simulink model "sim_SS_H2DF_2024a_GRU"  (R2024a)
settings: Solver=FixedStepAuto  StartTime=0.0  StopTime=4899  FixedStep=1  RelTol=1e-3  EnableMultiTasking=on
model workspace (MAT data in the model file):
  enable_IMEP_noise = 100
  enable_IMEP_offset = 1
values from neighbouring files (symbols this model uses):
  C2C_NMPC = init_C2C_NMPC_H2DF(C2C_NMPC.expdata)    [run_SS_H2DF_control.m]
undefined symbols (not defined in the file or in its folder): cost_length, horizon_length, y_ref_buf
libraries: matrix_library x3
(part 1 of 3)
settings Model: ExtModeTrigDuration=2  Creator=maxim  LastModifiedBy=winkler_a
settings SolverCC: PositivePriorityOrder=on
settings OptimizationCC: DefaultParameterBehavior=Inlined  EnhancedBackFolding=on  PassReuseOutputArgsAs=Individual arguments  ZeroExternalMemoryAtStartup=off  ZeroInternalMemoryAtStartup=off  MaxStackSize=64  OptimizeBlockOrder=speed  DifferentSizesBufferReuse=on  OptimizationCustomize=off  EfficientTunableParamExpr=on
settings DebuggingCC: ParameterTunabilityLossMsg=error
settings HardwareCC: ProdBitPerPointer=32  ProdBitPerSizeT=32  ProdBitPerPtrDiffT=32  ProdLargestAtomicInteger=Long  ProdLargestAtomicFloat=Double  ProdWordSize=32  ProdLongLongMode=on  ProdHWDeviceType=ARM Compatible->ARM Cortex
settings SFSimCC: SimUserSources=C2C_NMPC_model/C2C_NMPC_dyn_disc_phi_fun.c C2C_NMPC_model/C2C_NMPC_dyn_disc_phi_fun_jac.c C2C_NMPC_constraints/C2C_NMPC_constr_h_fun.c C2C_NMPC_constraints/C2C_NMPC_constr_h_fun_jac_uxt_zt.c C2C_NMPC_constraints/C2C_NMPC_constr_h_e_fun.c C2C_NMPC_constraints/C2C_NMPC_constr_h_e_fun_jac_uxt_zt.c acados_solver_sfunction_C2C_NMPC.c acados_solver_C2C_NMPC.c
settings SFSimCC: SimUserIncludeDirs=|
  | /include
  | /include/acados_c
  | /include/blasfeo/include
  | /include/hpipm/include
  | /lib
  | /c_generated_code
settings SFSimCC: SimUserLibraries=|
  | lib/libblasfeo.so
  | lib/libacados.so
  | lib/libhpipm.so
settings RTWCC: Description=Embedded Coder  SystemTargetFile=ert.tlc  TemplateMakefile=ert_default_tmf  RTWUseSimCustomCode=on  CustomSource=C2C_NMPC_model/C2C_NMPC_dyn_disc_phi_fun.c C2C_NMPC_model/C2C_NMPC_dyn_disc_phi_fun_jac.c C2C_NMPC_constraints/C2C_NMPC_constr_h_fun.c C2C_NMPC_constraints/C2C_NMPC_constr_h_fun_jac_uxt_zt.c C2C_NMPC_constraints/C2C_NMPC_constr_h_e_fun.c C2C_NMPC_constraints/C2C_NMPC_constr_h_e_fun_jac_uxt_zt.c acados_solver_sfunction_C2C_NMPC.c acados_solver_C2C_NMPC.c  Toolchain=GNU GCC Embedded Linux  BuildConfiguration=Faster Runs  GPUComputeCapability=3.5
settings RTWCC: CustomInclude=|
  | /include
  | /include/acados_c
  | /include/blasfeo/include
  | /include/hpipm/include
  | /lib
  | /c_generated_code
settings RTWCC: CustomLibrary=|
  | lib/libblasfeo.so
  | lib/libacados.so
  | lib/libhpipm.so
settings CodeAppCC: ForceParamTrailComments=on  IgnoreCustomStorageClasses=off  OperatorAnnotations=on  SimulinkDataObjDesc=on  SFDataObjDesc=on  InsertBlockDesc=on
settings ERTTargetCC: SupportContinuousTime=on  SupportNonInlinedSFcns=on  SupportVariableSizeSignals=on  ERTCustomFileTemplate=example_file_process.tlc

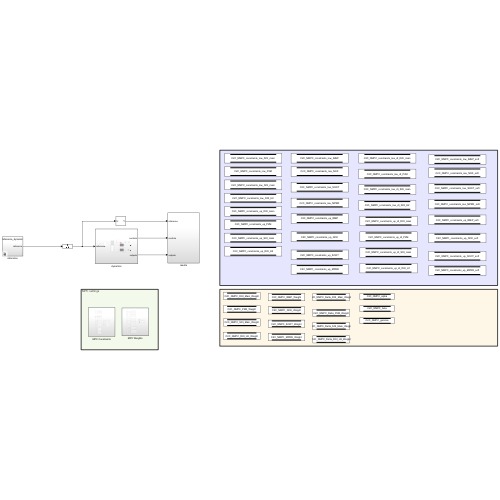
[thumbnail: Simulink's stored preview of the top-level diagram]
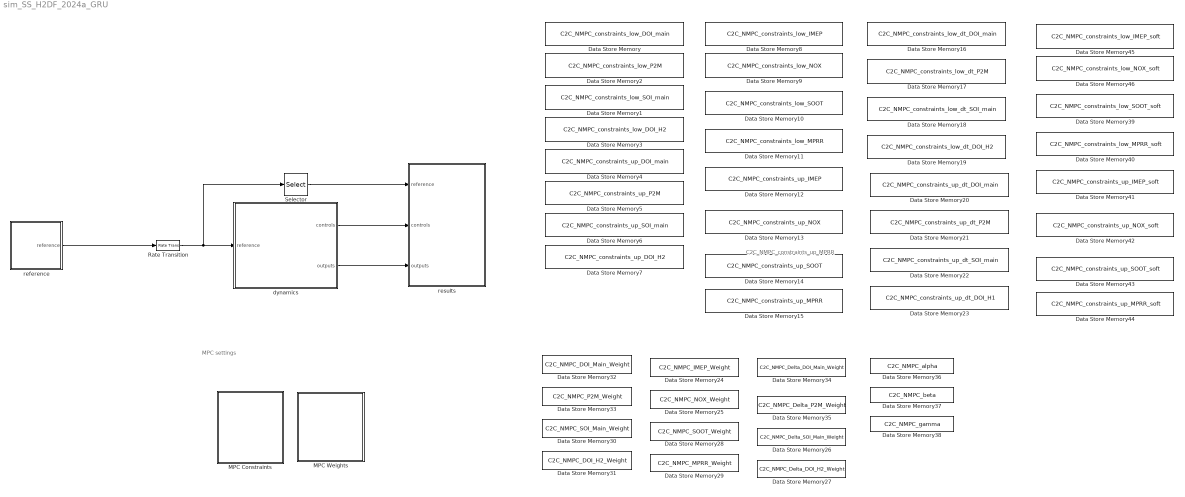
== system sim_SS_H2DF_2024a_GRU ==
  note: MPC settings
  note: C2C_NMPC_constraints_up_MPRR
  Data Store Memory : DataStoreMemory  DataStoreName=C2C_NMPC_constraints_low_DOI_main  WriteAfterWriteMsg=warning  ShowAdditionalParam=off
  Data Store Memory1 : DataStoreMemory  DataStoreName=C2C_NMPC_constraints_low_SOI_main  WriteAfterWriteMsg=warning  ShowAdditionalParam=off
  Data Store Memory10 : DataStoreMemory  DataStoreName=C2C_NMPC_constraints_low_SOOT  WriteAfterWriteMsg=warning  ShowAdditionalParam=off
  Data Store Memory11 : DataStoreMemory  DataStoreName=C2C_NMPC_constraints_low_MPRR  WriteAfterWriteMsg=warning  ShowAdditionalParam=off
  Data Store Memory12 : DataStoreMemory  DataStoreName=C2C_NMPC_constraints_up_IMEP  WriteAfterWriteMsg=warning  ShowAdditionalParam=off
  Data Store Memory13 : DataStoreMemory  DataStoreName=C2C_NMPC_constraints_up_NOX  WriteAfterWriteMsg=warning  ShowAdditionalParam=off
  Data Store Memory14 : DataStoreMemory  DataStoreName=C2C_NMPC_constraints_up_SOOT  WriteAfterWriteMsg=warning  ShowAdditionalParam=off
  Data Store Memory15 : DataStoreMemory  DataStoreName=C2C_NMPC_constraints_up_MPRR  WriteAfterWriteMsg=warning  ShowAdditionalParam=off
  Data Store Memory16 : DataStoreMemory  DataStoreName=C2C_NMPC_constraints_low_dt_DOI_main  WriteAfterWriteMsg=warning  ShowAdditionalParam=off
  Data Store Memory17 : DataStoreMemory  DataStoreName=C2C_NMPC_constraints_low_dt_P2M  WriteAfterWriteMsg=warning  ShowAdditionalParam=off
  Data Store Memory18 : DataStoreMemory  DataStoreName=C2C_NMPC_constraints_low_dt_SOI_main  WriteAfterWriteMsg=warning  ShowAdditionalParam=off
  Data Store Memory19 : DataStoreMemory  DataStoreName=C2C_NMPC_constraints_low_dt_DOI_H2  WriteAfterWriteMsg=warning  ShowAdditionalParam=off
  Data Store Memory2 : DataStoreMemory  DataStoreName=C2C_NMPC_constraints_low_P2M  WriteAfterWriteMsg=warning  ShowAdditionalParam=off
  Data Store Memory20 : DataStoreMemory  DataStoreName=C2C_NMPC_constraints_up_dt_DOI_main  WriteAfterWriteMsg=warning  ShowAdditionalParam=off
  Data Store Memory21 : DataStoreMemory  DataStoreName=C2C_NMPC_constraints_up_dt_P2M  WriteAfterWriteMsg=warning  ShowAdditionalParam=off
  Data Store Memory22 : DataStoreMemory  DataStoreName=C2C_NMPC_constraints_up_dt_SOI_main  WriteAfterWriteMsg=warning  ShowAdditionalParam=off
  Data Store Memory23 : DataStoreMemory  DataStoreName=C2C_NMPC_constraints_up_dt_DOI_H1  WriteAfterWriteMsg=warning  ShowAdditionalParam=off
  Data Store Memory24 : DataStoreMemory  DataStoreName=C2C_NMPC_IMEP_Weight  WriteAfterWriteMsg=warning  ShowAdditionalParam=off
  Data Store Memory25 : DataStoreMemory  DataStoreName=C2C_NMPC_NOX_Weight  WriteAfterWriteMsg=warning  ShowAdditionalParam=off
  Data Store Memory26 : DataStoreMemory  DataStoreName=C2C_NMPC_Delta_SOI_Main_Weight  WriteAfterWriteMsg=warning  ShowAdditionalParam=off
  Data Store Memory27 : DataStoreMemory  DataStoreName=C2C_NMPC_Delta_DOI_H2_Weight  WriteAfterWriteMsg=warning  ShowAdditionalParam=off
  Data Store Memory28 : DataStoreMemory  DataStoreName=C2C_NMPC_SOOT_Weight  WriteAfterWriteMsg=warning  ShowAdditionalParam=off
  Data Store Memory29 : DataStoreMemory  DataStoreName=C2C_NMPC_MPRR_Weight  WriteAfterWriteMsg=warning  ShowAdditionalParam=off
  Data Store Memory3 : DataStoreMemory  DataStoreName=C2C_NMPC_constraints_low_DOI_H2  WriteAfterWriteMsg=warning  ShowAdditionalParam=off
  Data Store Memory30 : DataStoreMemory  DataStoreName=C2C_NMPC_SOI_Main_Weight  WriteAfterWriteMsg=warning  ShowAdditionalParam=off
  Data Store Memory31 : DataStoreMemory  DataStoreName=C2C_NMPC_DOI_H2_Weight  WriteAfterWriteMsg=warning  ShowAdditionalParam=off
  Data Store Memory32 : DataStoreMemory  DataStoreName=C2C_NMPC_DOI_Main_Weight  WriteAfterWriteMsg=warning  ShowAdditionalParam=off
  Data Store Memory33 : DataStoreMemory  DataStoreName=C2C_NMPC_P2M_Weight  WriteAfterWriteMsg=warning  ShowAdditionalParam=off
  Data Store Memory34 : DataStoreMemory  DataStoreName=C2C_NMPC_Delta_DOI_Main_Weight  WriteAfterWriteMsg=warning  ShowAdditionalParam=off
  Data Store Memory35 : DataStoreMemory  DataStoreName=C2C_NMPC_Delta_P2M_Weight  WriteAfterWriteMsg=warning  ShowAdditionalParam=off
  Data Store Memory36 : DataStoreMemory  DataStoreName=C2C_NMPC_alpha  WriteAfterWriteMsg=warning  ShowAdditionalParam=off
  Data Store Memory37 : DataStoreMemory  DataStoreName=C2C_NMPC_beta  WriteAfterWriteMsg=warning  ShowAdditionalParam=off
  Data Store Memory38 : DataStoreMemory  DataStoreName=C2C_NMPC_gamma  WriteAfterWriteMsg=warning  ShowAdditionalParam=off
  Data Store Memory39 : DataStoreMemory  DataStoreName=C2C_NMPC_constraints_low_SOOT_soft  WriteAfterWriteMsg=warning  ShowAdditionalParam=off
  Data Store Memory4 : DataStoreMemory  DataStoreName=C2C_NMPC_constraints_up_DOI_main  WriteAfterWriteMsg=warning  ShowAdditionalParam=off
  Data Store Memory40 : DataStoreMemory  DataStoreName=C2C_NMPC_constraints_low_MPRR_soft  WriteAfterWriteMsg=warning  ShowAdditionalParam=off
  Data Store Memory41 : DataStoreMemory  DataStoreName=C2C_NMPC_constraints_up_IMEP_soft  WriteAfterWriteMsg=warning  ShowAdditionalParam=off
  Data Store Memory42 : DataStoreMemory  DataStoreName=C2C_NMPC_constraints_up_NOX_soft  WriteAfterWriteMsg=warning  ShowAdditionalParam=off
  Data Store Memory43 : DataStoreMemory  DataStoreName=C2C_NMPC_constraints_up_SOOT_soft  WriteAfterWriteMsg=warning  ShowAdditionalParam=off
  Data Store Memory44 : DataStoreMemory  DataStoreName=C2C_NMPC_constraints_up_MPRR_soft  WriteAfterWriteMsg=warning  ShowAdditionalParam=off
  Data Store Memory45 : DataStoreMemory  DataStoreName=C2C_NMPC_constraints_low_IMEP_soft  WriteAfterWriteMsg=warning  ShowAdditionalParam=off
  Data Store Memory46 : DataStoreMemory  DataStoreName=C2C_NMPC_constraints_low_NOX_soft  WriteAfterWriteMsg=warning  ShowAdditionalParam=off
  Data Store Memory5 : DataStoreMemory  DataStoreName=C2C_NMPC_constraints_up_P2M  WriteAfterWriteMsg=warning  ShowAdditionalParam=off
  Data Store Memory6 : DataStoreMemory  DataStoreName=C2C_NMPC_constraints_up_SOI_main  WriteAfterWriteMsg=warning  ShowAdditionalParam=off
  Data Store Memory7 : DataStoreMemory  DataStoreName=C2C_NMPC_constraints_up_DOI_H2  WriteAfterWriteMsg=warning  ShowAdditionalParam=off
  Data Store Memory8 : DataStoreMemory  DataStoreName=C2C_NMPC_constraints_low_IMEP  WriteAfterWriteMsg=warning  ShowAdditionalParam=off
  Data Store Memory9 : DataStoreMemory  DataStoreName=C2C_NMPC_constraints_low_NOX  WriteAfterWriteMsg=warning  ShowAdditionalParam=off
  MPC Constraints : Subsystem
  MPC Weights : Subsystem
  Rate Transition : RateTransition  Integrity=off  OutPortSampleTime=1
  Selector : Selector  InputPortWidth=C2C_NMPC.Dims.n_cost*3  IndexOptions=Index vector (dialog)  Indices=1:C2C_NMPC.Dims.n_cost  OutputSizes=1
  dynamics : Subsystem
  reference : Subsystem  Variant=on  VariantControlMode=label  VariantControl=Choice  LabelModeActiveChoice=reference_dynamic
  results : Subsystem
  wires:
  dynamics/2(outputs) -> results/3(outputs)
  Rate Transition/1 -> dynamics/1(reference), Selector/1
  dynamics/1(controls) -> results/2(controls)
  Selector/1 -> results/1(reference)
  reference/1(reference) -> Rate Transition/1

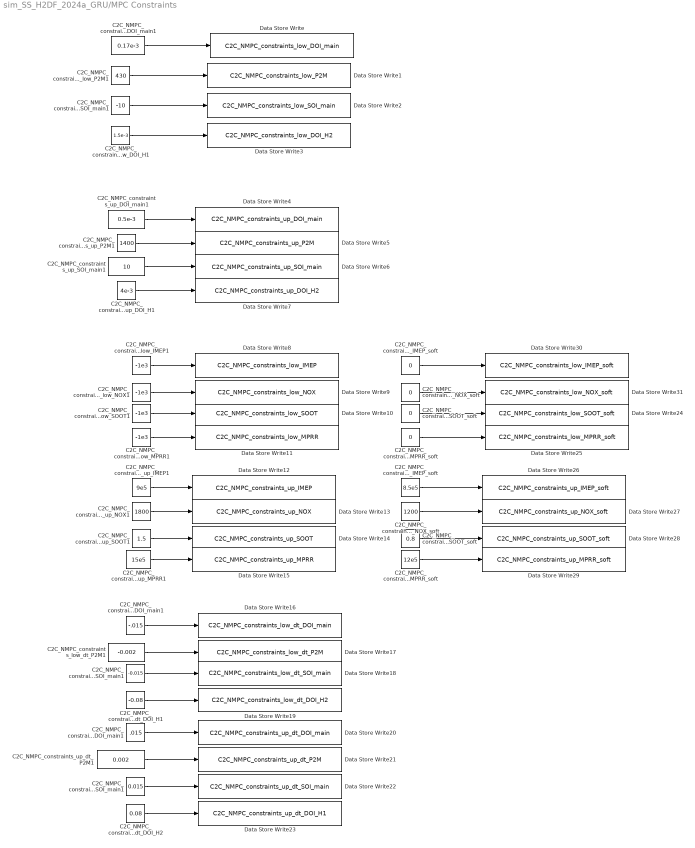
== system sim_SS_H2DF_2024a_GRU/MPC Constraints ==
  C2C_NMPC_constraints_low_DOI_H1 : Constant  Value=1.5e-3
  C2C_NMPC_constraints_low_DOI_main1 : Constant  Value=0.17e-3
  C2C_NMPC_constraints_low_IMEP1 : Constant  Value=-1e3
  C2C_NMPC_constraints_low_IMEP_soft : Constant  Value=0
  C2C_NMPC_constraints_low_MPRR1 : Constant  Value=-1e3
  C2C_NMPC_constraints_low_MPRR_soft : Constant  Value=0
  C2C_NMPC_constraints_low_NOX1 : Constant  Value=-1e3
  C2C_NMPC_constraints_low_NOX_soft : Constant  Value=0
  C2C_NMPC_constraints_low_P2M1 : Constant  Value=430
  C2C_NMPC_constraints_low_SOI_main1 : Constant  Value=-10
  C2C_NMPC_constraints_low_SOOT1 : Constant  Value=-1e3
  C2C_NMPC_constraints_low_SOOT_soft : Constant  Value=0
  C2C_NMPC_constraints_low_dt_DOI_H1 : Constant  Value=-0.08
  C2C_NMPC_constraints_low_dt_DOI_main1 : Constant  Value=-.015  VectorParams1D=off
  C2C_NMPC_constraints_low_dt_P2M1 : Constant  Value=-0.002
  C2C_NMPC_constraints_low_dt_SOI_main1 : Constant  Value=-0.015
  C2C_NMPC_constraints_up_DOI_H1 : Constant  Value=4e-3
  C2C_NMPC_constraints_up_DOI_main1 : Constant  Value=0.5e-3
  C2C_NMPC_constraints_up_IMEP1 : Constant  Value=9e5
  C2C_NMPC_constraints_up_IMEP_soft : Constant  Value=8.5e5
  C2C_NMPC_constraints_up_MPRR1 : Constant  Value=15e5
  C2C_NMPC_constraints_up_MPRR_soft : Constant  Value=12e5
  C2C_NMPC_constraints_up_NOX1 : Constant  Value=1800
  C2C_NMPC_constraints_up_NOX_soft : Constant  Value=1200
  C2C_NMPC_constraints_up_P2M1 : Constant  Value=1400
  C2C_NMPC_constraints_up_SOI_main1 : Constant  Value=10
  C2C_NMPC_constraints_up_SOOT1 : Constant  Value=1.5
  C2C_NMPC_constraints_up_SOOT_soft : Constant  Value=0.8
  C2C_NMPC_constraints_up_dt_DOI_H2 : Constant  Value=0.08
  C2C_NMPC_constraints_up_dt_DOI_main1 : Constant  Value=.015
  C2C_NMPC_constraints_up_dt_P2M1 : Constant  Value=0.002
  C2C_NMPC_constraints_up_dt_SOI_main1 : Constant  Value=0.015
  Data Store Write : DataStoreWrite  DataStoreName=C2C_NMPC_constraints_low_DOI_main  IndexOptions=Index vector (dialog)  Indices=1  OutputSizes=1
  Data Store Write1 : DataStoreWrite  DataStoreName=C2C_NMPC_constraints_low_P2M  IndexOptions=Index vector (dialog)  Indices=1  OutputSizes=1
  Data Store Write10 : DataStoreWrite  DataStoreName=C2C_NMPC_constraints_low_SOOT  IndexOptions=Index vector (dialog)  Indices=1  OutputSizes=1
  Data Store Write11 : DataStoreWrite  DataStoreName=C2C_NMPC_constraints_low_MPRR  IndexOptions=Index vector (dialog)  Indices=1  OutputSizes=1
  Data Store Write12 : DataStoreWrite  DataStoreName=C2C_NMPC_constraints_up_IMEP  IndexOptions=Index vector (dialog)  Indices=1  OutputSizes=1
  Data Store Write13 : DataStoreWrite  DataStoreName=C2C_NMPC_constraints_up_NOX  IndexOptions=Index vector (dialog)  Indices=1  OutputSizes=1
  Data Store Write14 : DataStoreWrite  DataStoreName=C2C_NMPC_constraints_up_SOOT  IndexOptions=Index vector (dialog)  Indices=1  OutputSizes=1
  Data Store Write15 : DataStoreWrite  DataStoreName=C2C_NMPC_constraints_up_MPRR  IndexOptions=Index vector (dialog)  Indices=1  OutputSizes=1
  Data Store Write16 : DataStoreWrite  DataStoreName=C2C_NMPC_constraints_low_dt_DOI_main  IndexOptions=Index vector (dialog)  Indices=1  OutputSizes=1
  Data Store Write17 : DataStoreWrite  DataStoreName=C2C_NMPC_constraints_low_dt_P2M  IndexOptions=Index vector (dialog)  Indices=1  OutputSizes=1
  Data Store Write18 : DataStoreWrite  DataStoreName=C2C_NMPC_constraints_low_dt_SOI_main  IndexOptions=Index vector (dialog)  Indices=1  OutputSizes=1
  Data Store Write19 : DataStoreWrite  DataStoreName=C2C_NMPC_constraints_low_dt_DOI_H2  IndexOptions=Index vector (dialog)  Indices=1  OutputSizes=1
  Data Store Write2 : DataStoreWrite  DataStoreName=C2C_NMPC_constraints_low_SOI_main  IndexOptions=Index vector (dialog)  Indices=1  OutputSizes=1
  Data Store Write20 : DataStoreWrite  DataStoreName=C2C_NMPC_constraints_up_dt_DOI_main  IndexOptions=Index vector (dialog)  Indices=1  OutputSizes=1
  Data Store Write21 : DataStoreWrite  DataStoreName=C2C_NMPC_constraints_up_dt_P2M  IndexOptions=Index vector (dialog)  Indices=1  OutputSizes=1
  Data Store Write22 : DataStoreWrite  DataStoreName=C2C_NMPC_constraints_up_dt_SOI_main  IndexOptions=Index vector (dialog)  Indices=1  OutputSizes=1
  Data Store Write23 : DataStoreWrite  DataStoreName=C2C_NMPC_constraints_up_dt_DOI_H1  IndexOptions=Index vector (dialog)  Indices=1  OutputSizes=1
  Data Store Write24 : DataStoreWrite  DataStoreName=C2C_NMPC_constraints_low_SOOT_soft  IndexOptions=Index vector (dialog)  Indices=1  OutputSizes=1
  Data Store Write25 : DataStoreWrite  DataStoreName=C2C_NMPC_constraints_low_MPRR_soft  IndexOptions=Index vector (dialog)  Indices=1  OutputSizes=1
  Data Store Write26 : DataStoreWrite  DataStoreName=C2C_NMPC_constraints_up_IMEP_soft  IndexOptions=Index vector (dialog)  Indices=1  OutputSizes=1
  Data Store Write27 : DataStoreWrite  DataStoreName=C2C_NMPC_constraints_up_NOX_soft  IndexOptions=Index vector (dialog)  Indices=1  OutputSizes=1
  Data Store Write28 : DataStoreWrite  DataStoreName=C2C_NMPC_constraints_up_SOOT_soft  IndexOptions=Index vector (dialog)  Indices=1  OutputSizes=1
  Data Store Write29 : DataStoreWrite  DataStoreName=C2C_NMPC_constraints_up_MPRR_soft  IndexOptions=Index vector (dialog)  Indices=1  OutputSizes=1
  Data Store Write3 : DataStoreWrite  DataStoreName=C2C_NMPC_constraints_low_DOI_H2  IndexOptions=Index vector (dialog)  Indices=1  OutputSizes=1
  Data Store Write30 : DataStoreWrite  DataStoreName=C2C_NMPC_constraints_low_IMEP_soft  IndexOptions=Index vector (dialog)  Indices=1  OutputSizes=1
  Data Store Write31 : DataStoreWrite  DataStoreName=C2C_NMPC_constraints_low_NOX_soft  IndexOptions=Index vector (dialog)  Indices=1  OutputSizes=1
  Data Store Write4 : DataStoreWrite  DataStoreName=C2C_NMPC_constraints_up_DOI_main  IndexOptions=Index vector (dialog)  Indices=1  OutputSizes=1
  Data Store Write5 : DataStoreWrite  DataStoreName=C2C_NMPC_constraints_up_P2M  IndexOptions=Index vector (dialog)  Indices=1  OutputSizes=1
  Data Store Write6 : DataStoreWrite  DataStoreName=C2C_NMPC_constraints_up_SOI_main  IndexOptions=Index vector (dialog)  Indices=1  OutputSizes=1
  Data Store Write7 : DataStoreWrite  DataStoreName=C2C_NMPC_constraints_up_DOI_H2  IndexOptions=Index vector (dialog)  Indices=1  OutputSizes=1
  Data Store Write8 : DataStoreWrite  DataStoreName=C2C_NMPC_constraints_low_IMEP  IndexOptions=Index vector (dialog)  Indices=1  OutputSizes=1
  Data Store Write9 : DataStoreWrite  DataStoreName=C2C_NMPC_constraints_low_NOX  IndexOptions=Index vector (dialog)  Indices=1  OutputSizes=1
  wires:
  C2C_NMPC_constraints_up_NOX1/1 -> Data Store Write13/1
  C2C_NMPC_constraints_up_dt_P2M1/1 -> Data Store Write21/1
  C2C_NMPC_constraints_low_dt_SOI_main1/1 -> Data Store Write18/1
  C2C_NMPC_constraints_up_dt_DOI_main1/1 -> Data Store Write20/1
  C2C_NMPC_constraints_low_dt_P2M1/1 -> Data Store Write17/1
  C2C_NMPC_constraints_up_dt_SOI_main1/1 -> Data Store Write22/1
  C2C_NMPC_constraints_up_DOI_main1/1 -> Data Store Write4/1
  C2C_NMPC_constraints_low_SOI_main1/1 -> Data Store Write2/1
  C2C_NMPC_constraints_up_P2M1/1 -> Data Store Write5/1
  C2C_NMPC_constraints_up_IMEP1/1 -> Data Store Write12/1
  C2C_NMPC_constraints_low_P2M1/1 -> Data Store Write1/1
  C2C_NMPC_constraints_up_SOOT1/1 -> Data Store Write14/1
  C2C_NMPC_constraints_up_MPRR1/1 -> Data Store Write15/1
  C2C_NMPC_constraints_low_dt_DOI_main1/1 -> Data Store Write16/1
  C2C_NMPC_constraints_low_DOI_main1/1 -> Data Store Write/1
  C2C_NMPC_constraints_low_dt_DOI_H1/1 -> Data Store Write19/1
  C2C_NMPC_constraints_low_MPRR1/1 -> Data Store Write11/1
  C2C_NMPC_constraints_low_DOI_H1/1 -> Data Store Write3/1
  C2C_NMPC_constraints_low_NOX1/1 -> Data Store Write9/1
  C2C_NMPC_constraints_low_IMEP1/1 -> Data Store Write8/1
  C2C_NMPC_constraints_up_SOI_main1/1 -> Data Store Write6/1
  C2C_NMPC_constraints_low_SOOT1/1 -> Data Store Write10/1
  C2C_NMPC_constraints_up_dt_DOI_H2/1 -> Data Store Write23/1
  C2C_NMPC_constraints_up_DOI_H1/1 -> Data Store Write7/1
  C2C_NMPC_constraints_low_SOOT_soft/1 -> Data Store Write24/1
  C2C_NMPC_constraints_low_IMEP_soft/1 -> Data Store Write30/1
  C2C_NMPC_constraints_low_NOX_soft/1 -> Data Store Write31/1
  C2C_NMPC_constraints_low_MPRR_soft/1 -> Data Store Write25/1
  C2C_NMPC_constraints_up_MPRR_soft/1 -> Data Store Write29/1
  C2C_NMPC_constraints_up_SOOT_soft/1 -> Data Store Write28/1
  C2C_NMPC_constraints_up_IMEP_soft/1 -> Data Store Write26/1
  C2C_NMPC_constraints_up_NOX_soft/1 -> Data Store Write27/1

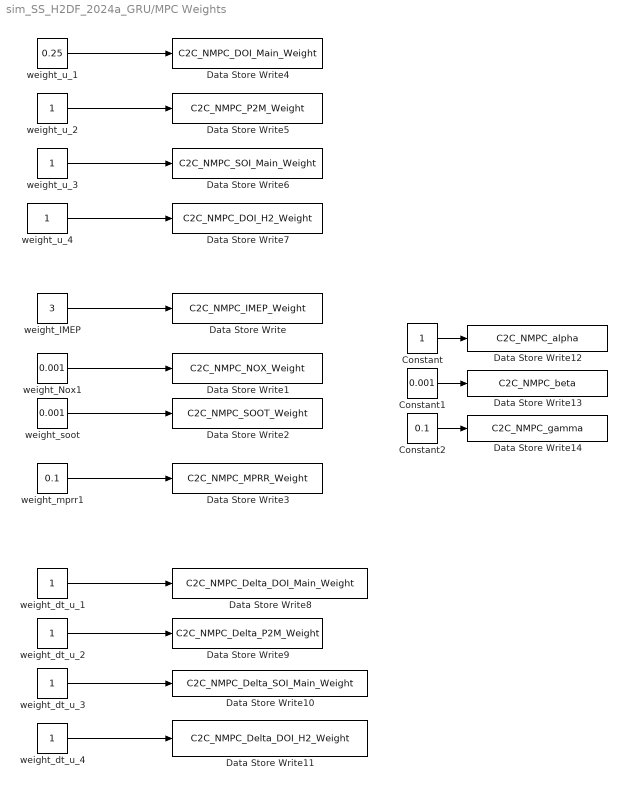
== system sim_SS_H2DF_2024a_GRU/MPC Weights ==
  Constant : Constant
  Constant1 : Constant  Value=0.001
  Constant2 : Constant  Value=0.1
  Data Store Write : DataStoreWrite  DataStoreName=C2C_NMPC_IMEP_Weight  IndexOptions=Index vector (dialog)  Indices=1  OutputSizes=1
  Data Store Write1 : DataStoreWrite  DataStoreName=C2C_NMPC_NOX_Weight  IndexOptions=Index vector (dialog)  Indices=1  OutputSizes=1
  Data Store Write10 : DataStoreWrite  DataStoreName=C2C_NMPC_Delta_SOI_Main_Weight  IndexOptions=Index vector (dialog)  Indices=1  OutputSizes=1
  Data Store Write11 : DataStoreWrite  DataStoreName=C2C_NMPC_Delta_DOI_H2_Weight  IndexOptions=Index vector (dialog)  Indices=1  OutputSizes=1
  Data Store Write12 : DataStoreWrite  DataStoreName=C2C_NMPC_alpha  IndexOptions=Index vector (dialog)  Indices=1  OutputSizes=1
  Data Store Write13 : DataStoreWrite  DataStoreName=C2C_NMPC_beta  IndexOptions=Index vector (dialog)  Indices=1  OutputSizes=1
  Data Store Write14 : DataStoreWrite  DataStoreName=C2C_NMPC_gamma  IndexOptions=Index vector (dialog)  Indices=1  OutputSizes=1
  Data Store Write2 : DataStoreWrite  DataStoreName=C2C_NMPC_SOOT_Weight  IndexOptions=Index vector (dialog)  Indices=1  OutputSizes=1
  Data Store Write3 : DataStoreWrite  DataStoreName=C2C_NMPC_MPRR_Weight  IndexOptions=Index vector (dialog)  Indices=1  OutputSizes=1
  Data Store Write4 : DataStoreWrite  DataStoreName=C2C_NMPC_DOI_Main_Weight  IndexOptions=Index vector (dialog)  Indices=1  OutputSizes=1
  Data Store Write5 : DataStoreWrite  DataStoreName=C2C_NMPC_P2M_Weight  IndexOptions=Index vector (dialog)  Indices=1  OutputSizes=1
  Data Store Write6 : DataStoreWrite  DataStoreName=C2C_NMPC_SOI_Main_Weight  IndexOptions=Index vector (dialog)  Indices=1  OutputSizes=1
  Data Store Write7 : DataStoreWrite  DataStoreName=C2C_NMPC_DOI_H2_Weight  IndexOptions=Index vector (dialog)  Indices=1  OutputSizes=1
  Data Store Write8 : DataStoreWrite  DataStoreName=C2C_NMPC_Delta_DOI_Main_Weight  IndexOptions=Index vector (dialog)  Indices=1  OutputSizes=1
  Data Store Write9 : DataStoreWrite  DataStoreName=C2C_NMPC_Delta_P2M_Weight  IndexOptions=Index vector (dialog)  Indices=1  OutputSizes=1
  weight_IMEP : Constant  Value=3
  weight_Nox1 : Constant  Value=0.001
  weight_dt_u_{1..4} (4 alike) : Constant
  weight_mprr1 : Constant  Value=0.1
  weight_soot : Constant  Value=0.001
  weight_u_1 : Constant  Value=0.25
  weight_u_2 : Constant
  weight_u_3 : Constant
  weight_u_4 : Constant
  wires:
  weight_soot/1 -> Data Store Write2/1
  weight_dt_u_4/1 -> Data Store Write11/1
  weight_dt_u_1/1 -> Data Store Write8/1
  weight_mprr1/1 -> Data Store Write3/1
  weight_dt_u_3/1 -> Data Store Write10/1
  weight_dt_u_2/1 -> Data Store Write9/1
  weight_Nox1/1 -> Data Store Write1/1
  weight_u_3/1 -> Data Store Write6/1
  weight_u_4/1 -> Data Store Write7/1
  weight_u_1/1 -> Data Store Write4/1
  weight_IMEP/1 -> Data Store Write/1
  weight_u_2/1 -> Data Store Write5/1
  Constant/1 -> Data Store Write12/1
  Constant2/1 -> Data Store Write14/1
  Constant1/1 -> Data Store Write13/1

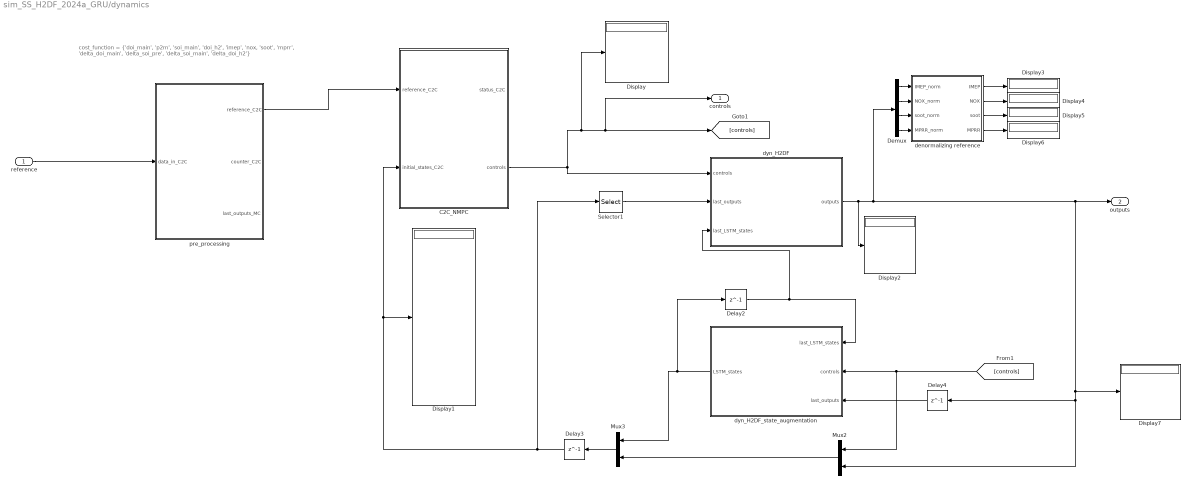
== system sim_SS_H2DF_2024a_GRU/dynamics ==
  note: cost_function = {'doi_main', 'p2m', 'soi_main', 'doi_h2', 'imep', 'nox, 'soot', 'mprr', 'delta_doi_main', 'delta_soi_pre', 'delta_soi_main', 'delta_doi_h2'}
  reference : Inport
  C2C_NMPC : Subsystem  Variant=on  VariantControlMode=label  VariantControl=Choice  LabelModeActiveChoice=C2C_NMPC_n3
  Delay2 : Delay  DelayLength=1  InitialCondition=C2C_NMPC.x0(1:C2C_NMPC.Dims.n_LSTM_states)
  Delay3 : Delay  DelayLength=1  InitialCondition=C2C_NMPC.x0
  Delay4 : Delay  DelayLength=1  InitialCondition=C2C_NMPC.x0((C2C_NMPC.Dims.n_states - C2C_NMPC.Dims.n_outputs + 1):C2C_NMPC.Dims.n_states)
  Demux : Demux
  Display{,1..7} (8 alike) : Display
  Mux2 : Mux  Inputs=2
  Mux3 : Mux  Inputs=2
  Selector1 : Selector  IndexOptions=Index vector (dialog)  Indices=[(C2C_NMPC.Dims.n_states - C2C_NMPC.Dims.n_outputs + 1):C2C_NMPC.Dims.n_states]  OutputSizes=1
  denormalizing reference : Subsystem
  dyn_H2DF : Subsystem  Variant=on  VariantControlMode=label  VariantControl=Choice  LabelModeActiveChoice=dyn_H2DF
  dyn_H2DF_state_augmentation : Subsystem  Variant=on  VariantControlMode=label  VariantControl=Choice  LabelModeActiveChoice=dyn_H2DF
  pre_processing : Subsystem
  controls : Outport
  outputs : Outport  Port=2
  wires:
  Delay3/1 -> Selector1/1, C2C_NMPC/2(initial_states_C2C), Display1/1
  [controls] -> Mux2/1, dyn_H2DF_state_augmentation/2(controls)
  Mux3/1 -> Delay3/1
  Mux2/1 -> Mux3/2
  Delay2/1 -> dyn_H2DF_state_augmentation/1(last_LSTM_states), dyn_H2DF/3(last_LSTM_states)
  reference/1 -> pre_processing/1(data_in_C2C)
  pre_processing/1(reference_C2C) -> C2C_NMPC/1(reference_C2C)
  dyn_H2DF/1(outputs) -> Display2/1, Delay4/1, Mux2/2, Display7/1, outputs/1, Demux/1
  Selector1/1 -> dyn_H2DF/2(last_outputs)
  Delay4/1 -> dyn_H2DF_state_augmentation/3(last_outputs)
  dyn_H2DF_state_augmentation/1(LSTM_states) -> Mux3/1, Delay2/1
  Demux/2 -> denormalizing reference/2(NOX_norm)
  Demux/1 -> denormalizing reference/1(IMEP_norm)
  Demux/3 -> denormalizing reference/3(soot_norm)
  Demux/4 -> denormalizing reference/4(MPRR_norm)
  denormalizing reference/1(IMEP) -> Display3/1
  denormalizing reference/4(MPRR) -> Display6/1
  denormalizing reference/3(soot) -> Display5/1
  denormalizing reference/2(NOX) -> Display4/1
  C2C_NMPC/2(controls) -> dyn_H2DF/1(controls), controls/1, [controls], Display/1

== system sim_SS_H2DF_2024a_GRU/reference ==
  note: ref is hardcoded for N=3 now
  reference_dynamic : Subsystem  Variant=on  VariantControlMode=label  VariantControl=reference_dynamic  LabelModeActiveChoice=Choice_1
  reference_static : Subsystem  VariantControl=reference_static
  reference : Outport

== system sim_SS_H2DF_2024a_GRU/results ==
  reference : Inport
  controls : Inport  Port=2
  outputs : Inport  Port=3
  Demux{1..4} (4 alike) : Demux
  Mux{1..3,7} (4 alike) : Mux  Inputs=2
  Mux6 : Mux
  Scope : Scope  NumInputPorts=8
  Selector5 : Selector  IndexOptions=Index vector (dialog)  Indices=[(C2C_NMPC.Dims.n_controls + 1 ):(C2C_NMPC.Dims.n_cost - C2C_NMPC.Dims.n_controls)]  OutputSizes=1
  To Workspace : ToWorkspace  VariableName=IMEP  SampleTime=-1
  To Workspace1 : ToWorkspace  VariableName=NOX  SampleTime=-1
  To Workspace2 : ToWorkspace  VariableName=soot  SampleTime=-1
  To Workspace3 : ToWorkspace  VariableName=MPRR  SampleTime=-1
  To Workspace4 : ToWorkspace  VariableName=DOI_main  SampleTime=-1
  To Workspace5 : ToWorkspace  VariableName=SOI_pre  SampleTime=-1
  To Workspace6 : ToWorkspace  VariableName=SOI_main  SampleTime=-1
  To Workspace7 : ToWorkspace  VariableName=DOI_H2  SampleTime=-1
  denormalizing physical controls and outputs : Subsystem
  denormalizing reference : Subsystem
  wires:
  reference/1 -> Selector5/1
  Selector5/1 -> Demux3/1
  outputs/1 -> Demux1/1
  controls/1 -> Demux2/1
  Mux7/1 -> To Workspace/1, Scope/1
  Mux2/1 -> To Workspace1/1, Scope/2
  Demux3/1 -> Mux7/1
  Mux3/1 -> To Workspace3/1, Scope/4
  Mux1/1 -> To Workspace2/1, Scope/3
  Demux4/2 -> To Workspace5/1, Scope/6
  Demux4/3 -> To Workspace6/1, Scope/7
  Demux4/1 -> To Workspace4/1, Scope/5
  Mux6/1 -> Demux4/1
  Demux1/1 -> denormalizing physical controls and outputs/1(IMEP_norm)
  Demux1/2 -> denormalizing physical controls and outputs/2(NOX_norm)
  Demux1/3 -> denormalizing physical controls and outputs/3(soot_norm)
  Demux1/4 -> denormalizing physical controls and outputs/4(MPRR_norm)
  Demux2/1 -> denormalizing physical controls and outputs/5(DOI_main_norm)
  Demux2/2 -> denormalizing physical controls and outputs/6(SOI_pre_norm)
  Demux2/3 -> denormalizing physical controls and outputs/7(SOI_main_norm)
  denormalizing physical controls and outputs/1(IMEP) -> Mux7/2
  denormalizing physical controls and outputs/5(DOI_main) -> Mux6/1
  denormalizing physical controls and outputs/6(SOI_pre) -> Mux6/2
  denormalizing physical controls and outputs/7(SOI_main) -> Mux6/3
  Demux3/3 -> Mux1/1
  Demux3/4 -> Mux3/1
  denormalizing physical controls and outputs/2(NOX) -> Mux2/2
  denormalizing physical controls and outputs/3(soot) -> Mux1/2
  denormalizing physical controls and outputs/4(MPRR) -> Mux3/2
  Demux2/4 -> denormalizing physical controls and outputs/8(DOI_H2_norm)
  denormalizing physical controls and outputs/8(DOI_H2) -> Mux6/4
  Demux4/4 -> To Workspace7/1, Scope/8
  Demux3/2 -> Mux2/1

== system sim_SS_H2DF_2024a_GRU/dynamics/C2C_NMPC ==
  reference_C2C : Inport
  initial_states_C2C : Inport  Port=2
  C2C_NMPC_n3 : Subsystem  VariantControl=C2C_NMPC_n3
  status_C2C : Outport
  controls : Outport  Port=2

== system sim_SS_H2DF_2024a_GRU/dynamics/denormalizing reference ==
  IMEP_norm : Inport
  NOX_norm : Inport  Port=2
  soot_norm : Inport  Port=3
  MPRR_norm : Inport  Port=4
  Constant : Constant  Value=C2C_NMPC.Normalization.outputs.mean(1)
  Constant1 : Constant  Value=C2C_NMPC.Normalization.outputs.mean(2)
  Constant2 : Constant  Value=C2C_NMPC.Normalization.outputs.mean(3)
  Constant3 : Constant  Value=C2C_NMPC.Normalization.outputs.mean(4)
  Gain : Gain  Gain=C2C_NMPC.Normalization.outputs.std(1)
  Gain1 : Gain  Gain=C2C_NMPC.Normalization.outputs.std(2)
  Gain2 : Gain  Gain=C2C_NMPC.Normalization.outputs.std(3)
  Gain3 : Gain  Gain=C2C_NMPC.Normalization.outputs.std(4)
  Sum{1..3,5} (4 alike) : Sum  Inputs=|++
  IMEP : Outport
  NOX : Outport  Port=2
  soot : Outport  Port=3
  MPRR : Outport  Port=4
  wires:
  Gain/1 -> Sum5/1
  IMEP_norm/1 -> Gain/1
  Constant/1 -> Sum5/2
  Sum5/1 -> IMEP/1
  Gain1/1 -> Sum1/1
  Constant1/1 -> Sum1/2
  NOX_norm/1 -> Gain1/1
  Sum1/1 -> NOX/1
  Gain2/1 -> Sum2/1
  Constant2/1 -> Sum2/2
  soot_norm/1 -> Gain2/1
  Sum2/1 -> soot/1
  Gain3/1 -> Sum3/1
  Constant3/1 -> Sum3/2
  MPRR_norm/1 -> Gain3/1
  Sum3/1 -> MPRR/1

== system sim_SS_H2DF_2024a_GRU/dynamics/dyn_H2DF ==
  controls : Inport  PortDimensions=C2C_NMPC.Dims.n_controls
  last_outputs : Inport  Port=2
  last_LSTM_states : Inport  Port=3
  dyn_H2DF : Subsystem  VariantControl=dyn_H2DF
  dyn_H2DF_nofb : Subsystem  VariantControl=dyn_H2DF_nofb
  outputs : Outport

== system sim_SS_H2DF_2024a_GRU/dynamics/dyn_H2DF_state_augmentation ==
  last_LSTM_states : Inport
  controls : Inport  Port=2
  last_outputs : Inport  Port=3
  dyn_H2DF_state_augmentation : Subsystem  VariantControl=dyn_H2DF
  dyn_H2DF_state_augmentation_nofb : Subsystem  VariantControl=dyn_H2DF_nofb
  LSTM_states : Outport

== system sim_SS_H2DF_2024a_GRU/dynamics/pre_processing ==
  data_in_C2C : Inport
  Selector : Selector  IndexOptions=Index vector (dialog)  Indices=[6]  OutputSizes=1
  normalize_last_outputs_MC : Subsystem
  normalize_reference_C2C : Subsystem
  reference_C2C : Outport  VectorParamsAs1DForOutWhenUnconnected=off
  counter_C2C : Outport  Port=2  VectorParamsAs1DForOutWhenUnconnected=off
  last_outputs_MC : Outport  Port=3  VectorParamsAs1DForOutWhenUnconnected=off
  wires:
  normalize_reference_C2C/1(reference_C2C) -> reference_C2C/1
  data_in_C2C/1 -> Selector/1, normalize_last_outputs_MC/1(data_in), normalize_reference_C2C/1(data_in)
  normalize_last_outputs_MC/1(last_outputs_MC) -> last_outputs_MC/1
  Selector/1 -> counter_C2C/1

== system sim_SS_H2DF_2024a_GRU/reference/reference_dynamic ==
  reference_dynamic : Subsystem  VariantControl=Choice_1
  reference : Outport

== system sim_SS_H2DF_2024a_GRU/reference/reference_static ==
  Add1 : Sum
  Clock : Clock
  Constant : Constant
  Constant1 : Constant  Value=[C2C_NMPC.controls_ref;C2C_NMPC.outputs_ref; zeros(C2C_NMPC.Dims.n_controls, length(C2C_NMPC.controls_ref(1, :)))]
  Mux : Mux  Inputs=3
  ref_func : MATLAB Function  TreatAsAtomicUnit=on
  reference : Outport  VectorParamsAs1DForOutWhenUnconnected=off
  wires:
  Constant1/1 -> ref_func/1(ref_norm)
  Constant/1 -> Add1/2
  Add1/1 -> ref_func/2(init_index)
  Clock/1 -> Add1/1
  Mux/1 -> reference/1
  ref_func/1(y_ref) -> Mux/3, Mux/1, Mux/2

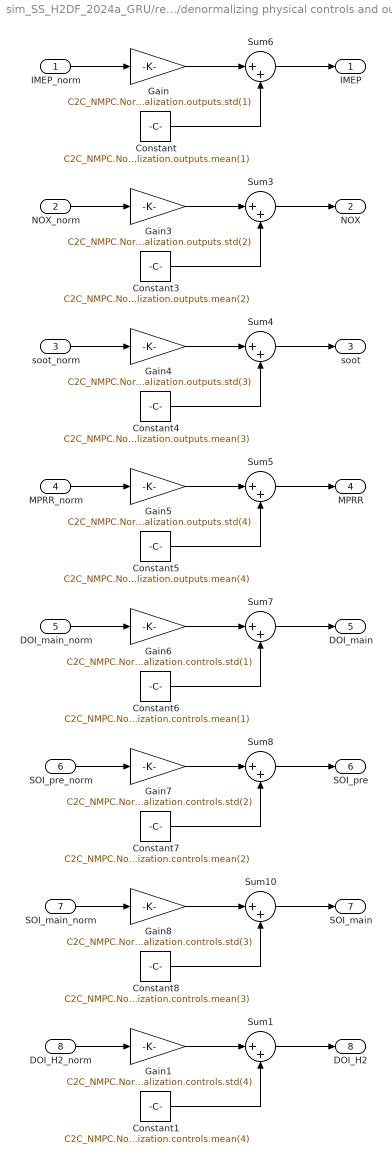
== system sim_SS_H2DF_2024a_GRU/results/denormalizing physical controls and outputs ==
  IMEP_norm : Inport
  NOX_norm : Inport  Port=2
  soot_norm : Inport  Port=3
  MPRR_norm : Inport  Port=4
  DOI_main_norm : Inport  Port=5
  SOI_pre_norm : Inport  Port=6
  SOI_main_norm : Inport  Port=7
  DOI_H2_norm : Inport  Port=8
  Constant : Constant  Value=C2C_NMPC.Normalization.outputs.mean(1)
  Constant1 : Constant  Value=C2C_NMPC.Normalization.controls.mean(4)
  Constant3 : Constant  Value=C2C_NMPC.Normalization.outputs.mean(2)
  Constant4 : Constant  Value=C2C_NMPC.Normalization.outputs.mean(3)
  Constant5 : Constant  Value=C2C_NMPC.Normalization.outputs.mean(4)
  Constant6 : Constant  Value=C2C_NMPC.Normalization.controls.mean(1)
  Constant7 : Constant  Value=C2C_NMPC.Normalization.controls.mean(2)
  Constant8 : Constant  Value=C2C_NMPC.Normalization.controls.mean(3)
  Gain : Gain  Gain=C2C_NMPC.Normalization.outputs.std(1)
  Gain1 : Gain  Gain=C2C_NMPC.Normalization.controls.std(4)
  Gain3 : Gain  Gain=C2C_NMPC.Normalization.outputs.std(2)
  Gain4 : Gain  Gain=C2C_NMPC.Normalization.outputs.std(3)
  Gain5 : Gain  Gain=C2C_NMPC.Normalization.outputs.std(4)
  Gain6 : Gain  Gain=C2C_NMPC.Normalization.controls.std(1)
  Gain7 : Gain  Gain=C2C_NMPC.Normalization.controls.std(2)
  Gain8 : Gain  Gain=C2C_NMPC.Normalization.controls.std(3)
  Sum{1,3..8,10} (8 alike) : Sum  Inputs=|++
  IMEP : Outport
  NOX : Outport  Port=2
  soot : Outport  Port=3
  MPRR : Outport  Port=4
  DOI_main : Outport  Port=5
  SOI_pre : Outport  Port=6
  SOI_main : Outport  Port=7
  DOI_H2 : Outport  Port=8
  wires:
  Gain4/1 -> Sum4/1
  Constant3/1 -> Sum3/2
  Constant4/1 -> Sum4/2
  Gain3/1 -> Sum3/1
  Constant5/1 -> Sum5/2
  Gain5/1 -> Sum5/1
  Constant/1 -> Sum6/2
  Sum3/1 -> NOX/1
  NOX_norm/1 -> Gain3/1
  Sum5/1 -> MPRR/1
  Gain/1 -> Sum6/1
  IMEP_norm/1 -> Gain/1
  Sum6/1 -> IMEP/1
  MPRR_norm/1 -> Gain5/1
  Sum4/1 -> soot/1
  soot_norm/1 -> Gain4/1
  Constant7/1 -> Sum8/2
  Gain8/1 -> Sum10/1
  Constant6/1 -> Sum7/2
  Gain7/1 -> Sum8/1
  Sum10/1 -> SOI_main/1
  DOI_main_norm/1 -> Gain6/1
  Sum7/1 -> DOI_main/1
  Gain6/1 -> Sum7/1
  Sum8/1 -> SOI_pre/1
  Constant8/1 -> Sum10/2
  SOI_main_norm/1 -> Gain8/1
  SOI_pre_norm/1 -> Gain7/1
  DOI_H2_norm/1 -> Gain1/1
  Constant1/1 -> Sum1/2
  Gain1/1 -> Sum1/1
  Sum1/1 -> DOI_H2/1

== system sim_SS_H2DF_2024a_GRU/results/denormalizing reference ==
  IMEP_norm : Inport
  NOX_norm : Inport  Port=2
  soot_norm : Inport  Port=3
  MPRR_norm : Inport  Port=4
  Constant : Constant  Value=C2C_NMPC.Normalization.outputs.mean(1)
  Constant1 : Constant  Value=C2C_NMPC.Normalization.outputs.mean(2)
  Constant2 : Constant  Value=C2C_NMPC.Normalization.outputs.mean(3)
  Constant3 : Constant  Value=C2C_NMPC.Normalization.outputs.mean(4)
  Gain : Gain  Gain=C2C_NMPC.Normalization.outputs.std(1)
  Gain1 : Gain  Gain=C2C_NMPC.Normalization.outputs.std(2)
  Gain2 : Gain  Gain=C2C_NMPC.Normalization.outputs.std(3)
  Gain3 : Gain  Gain=C2C_NMPC.Normalization.outputs.std(4)
  Sum{1..3,5} (4 alike) : Sum  Inputs=|++
  IMEP : Outport
  NOX : Outport  Port=2
  soot : Outport  Port=3
  MPRR : Outport  Port=4
  wires:
  Gain/1 -> Sum5/1
  IMEP_norm/1 -> Gain/1
  Constant/1 -> Sum5/2
  Sum5/1 -> IMEP/1
  Gain1/1 -> Sum1/1
  Constant1/1 -> Sum1/2
  NOX_norm/1 -> Gain1/1
  Sum1/1 -> NOX/1
  Gain2/1 -> Sum2/1
  Constant2/1 -> Sum2/2
  soot_norm/1 -> Gain2/1
  Sum2/1 -> soot/1
  Gain3/1 -> Sum3/1
  Constant3/1 -> Sum3/2
  MPRR_norm/1 -> Gain3/1
  Sum3/1 -> MPRR/1

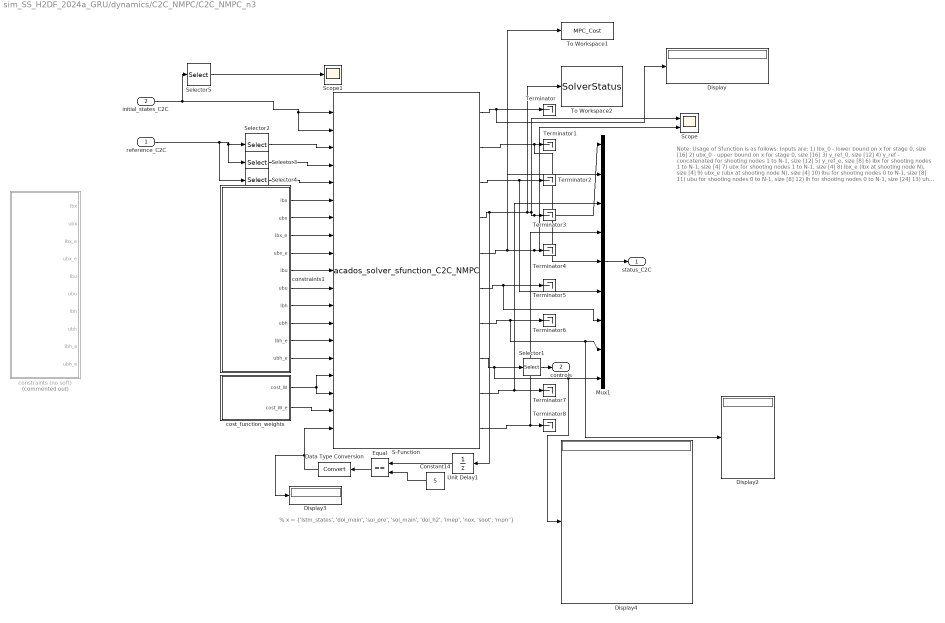
== system sim_SS_H2DF_2024a_GRU/dynamics/C2C_NMPC/C2C_NMPC_n3 ==
  note: Note: Usage of Sfunction is as follows:
      | Inputs are:
      | 1) lbx_0 - lower bound on x for stage 0, size [16]
      | 2) ubx_0 - upper bound on x for stage 0, size [16]
      | 3) y_ref_0, size [12]
      | 4) y_ref - concatenated for shooting nodes 1 to N-1, size [12]
      | 5) y_ref_e, size [8]
      | 6) lbx for shooting nodes 1 to N-1, size [4]
      | 7) ubx for shooting nodes 1 to N-1, size [4]
      | 8) lbx_e (lbx at shooting node N), size [4]
      | 9) ubx_e (ubx at shooting node N), size [4]
      | 10) lbu for shooting nodes 0 to N-1, size [8]
      | 11) ubu for shooting nodes 0 to N-1, size [8]
      | 12) lh for shooting nodes 0 to N-1, size [24]
      | 13) uh for shooting nodes 0 to N-1, size [24]
      | 14) lh_e, size [8]
      | 15) uh_e, size [8]
      | 16) cost_W_0 in column-major format, size [144]
      | 17) cost_W in column-major format, that is set for all intermediate shooting nodes: 1 to N-1, size [144]
      | 18) cost_W_e in column-major format, size [64]
      | 19) reset_solver determines if iterate is set to all zeros before other initializations (x_init, u_init) are set and before solver is called, size [1]
      |
      | Outputs are:
      | 1) u0, control input at node 0, size [4]
      | 2) utraj, control input concatenated for nodes 0 to N-1, size [8]
      | 3) xtraj, state concatenated for nodes 0 to N, size [48]
      | 4) acados solver status (0 = SUCCESS)
      | 5) cost function value
      | 6) KKT residual
      | 7) KKT residuals, size [4] (stat, eq, ineq, comp)
      | 8) x1, state at node 1
      | 9) CPU time
      | 10) SQP iterations
  note: % x = {'lstm_states', 'doi_main', 'soi_pre', 'soi_main', 'doi_h2', 'imep', 'nox, 'soot', 'mprr'}
  reference_C2C : Inport
  initial_states_C2C : Inport  Port=2
  Constant14 : Constant  Value=5
  Data Type Conversion : DataTypeConversion  SaturateOnIntegerOverflow=off  RndMeth=Floor
  Display{,2..4} (4 alike) : Display
  Equal : RelationalOperator  Operator===  OutDataTypeStr=boolean  RndMeth=Simplest  InputSameDT=off
  Mux1 : Mux  Inputs=9
  S-Function : S-Function  FunctionName=acados_solver_sfunction_C2C_NMPC  SFunctionDeploymentMode=off  EnableBusSupport=off
  Scope : Scope  NumInputPorts=2
  Scope1 : Scope
  Selector1 : Selector  IndexOptions=Index vector (dialog)  Indices=[(C2C_NMPC.Dims.n_LSTM_states + 1):(C2C_NMPC.Dims.n_LSTM_states + C2C_NMPC.Dims.n_controls)]  OutputSizes=1
  Selector2 : Selector  IndexOptions=Index vector (dialog)  Indices=[1:(C2C_NMPC.Dims.n_cost)]  OutputSizes=1
  Selector3 : Selector  IndexOptions=Index vector (dialog)  Indices=[ (C2C_NMPC.Dims.n_cost + 1) : (C2C_NMPC.Dims.n_cost * 3) ]  OutputSizes=1
  Selector4 : Selector  IndexOptions=Index vector (dialog)  Indices=[ (C2C_NMPC.Dims.n_cost * 2 + 1) : (C2C_NMPC.Dims.n_cost * 2 + C2C_NMPC.Dims.n_controls + C2C_NMPC.Dims.n_outputs ) ]  OutputSizes=1
  Selector5 : Selector  IndexOptions=Index vector (dialog)  Indices=13  OutputSizes=1
  Terminator{,1..8} (9 alike) : Terminator
  To Workspace1 : ToWorkspace  VariableName=MPC_Cost  SampleTime=-1
  To Workspace2 : ToWorkspace  VariableName=SolverStatus  SampleTime=1
  Unit Delay1 : UnitDelay  SampleTime=-1  HasFrameUpgradeWarning=on
  constraints (no soft) : Subsystem  Commented=on
  constraints1 : Subsystem
  cost_function_weights : Subsystem
  status_C2C : Outport
  controls : Outport  Port=2
  wires:
  constraints1/5(lbu) -> S-Function/10
  constraints1/6(ubu) -> S-Function/11
  constraints1/7(lbh) -> S-Function/12
  constraints1/8(ubh) -> S-Function/13
  constraints1/9(lbh_e) -> S-Function/14
  constraints1/10(ubh_e) -> S-Function/15
  cost_function_weights/1(cost_W) -> S-Function/16, S-Function/17
  Data Type Conversion/1 -> S-Function/19, Display3/1
  constraints1/1(lbx) -> S-Function/6
  constraints1/2(ubx) -> S-Function/7
  constraints1/3(lbx_e) -> S-Function/8
  constraints1/4(ubx_e) -> S-Function/9
  S-Function/5 -> To Workspace1/1, Terminator4/1, Scope/2, Mux1/2
  Equal/1 -> Data Type Conversion/1
  Unit Delay1/1 -> Equal/1
  Constant14/1 -> Equal/2
  Mux1/1 -> status_C2C/1
  Selector1/1 -> controls/1
  Selector4/1 -> S-Function/5
  reference_C2C/1 -> Selector4/1, Selector3/1, Selector2/1
  initial_states_C2C/1 -> Selector5/1, S-Function/2, S-Function/1
  S-Function/10 -> Terminator8/1, Mux1/4
  S-Function/9 -> Terminator7/1, Mux1/3
  S-Function/7 -> Terminator6/1, Display2/1, Mux1/8
  S-Function/6 -> Terminator5/1, Mux1/7
  S-Function/8 -> Selector1/1, Display4/1, Mux1/9
  S-Function/4 -> Unit Delay1/1, To Workspace2/1, Scope/1, Mux1/1, Terminator3/1
  S-Function/3 -> Terminator2/1, Mux1/6
  S-Function/2 -> Terminator1/1, Mux1/5
  S-Function/1 -> Display/1, Terminator/1
  Selector2/1 -> S-Function/3
  Selector3/1 -> S-Function/4
  cost_function_weights/2(cost_W_e) -> S-Function/18
  Selector5/1 -> Scope1/1

== system sim_SS_H2DF_2024a_GRU/dynamics/dyn_H2DF/dyn_H2DF ==
  controls : Inport
  last_outputs : Inport  Port=2
  last_LSTM_states : Inport  Port=3
  Terminator : Terminator
  dyn_H2DF : MATLAB Function  TreatAsAtomicUnit=on
  outputs : Outport
  wires:
  last_LSTM_states/1 -> dyn_H2DF/1(last_LSTM_states)
  dyn_H2DF/2(LSTM_states) -> Terminator/1
  controls/1 -> dyn_H2DF/2(controls)
  dyn_H2DF/1(outputs) -> outputs/1
  last_outputs/1 -> dyn_H2DF/3(last_outputs)

== system sim_SS_H2DF_2024a_GRU/dynamics/dyn_H2DF/dyn_H2DF_nofb ==
  controls : Inport
  last_outputs : Inport  Port=2
  last_LSTM_states : Inport  Port=3
  Terminator : Terminator
  Terminator1 : Terminator
  dyn_H2DF : MATLAB Function  TreatAsAtomicUnit=on
  outputs : Outport
  wires:
  dyn_H2DF/1(outputs) -> outputs/1
  controls/1 -> dyn_H2DF/2(controls)
  dyn_H2DF/2(LSTM_states) -> Terminator/1
  last_LSTM_states/1 -> dyn_H2DF/1(last_LSTM_states)
  last_outputs/1 -> Terminator1/1

== system sim_SS_H2DF_2024a_GRU/dynamics/dyn_H2DF_state_augmentation/dyn_H2DF_state_augmentation ==
  last_LSTM_states : Inport
  controls : Inport  Port=2
  last_outputs : Inport  Port=3
  dyn_H2DF_state_augmentation : MATLAB Function  TreatAsAtomicUnit=on
  LSTM_states : Outport
  wires:
  dyn_H2DF_state_augmentation/1(LSTM_states) -> LSTM_states/1
  last_outputs/1 -> dyn_H2DF_state_augmentation/3(last_outputs)
  last_LSTM_states/1 -> dyn_H2DF_state_augmentation/1(last_LSTM_states)
  controls/1 -> dyn_H2DF_state_augmentation/2(controls)

== system sim_SS_H2DF_2024a_GRU/dynamics/dyn_H2DF_state_augmentation/dyn_H2DF_state_augmentation_nofb ==
  last_LSTM_states : Inport
  controls : Inport  Port=2
  last_outputs : Inport  Port=3
  Terminator : Terminator
  dyn_H2DF_state_augmentation : MATLAB Function  TreatAsAtomicUnit=on
  LSTM_states : Outport
  wires:
  controls/1 -> dyn_H2DF_state_augmentation/2(controls)
  last_LSTM_states/1 -> dyn_H2DF_state_augmentation/1(last_LSTM_states)
  dyn_H2DF_state_augmentation/1(LSTM_states) -> LSTM_states/1
  last_outputs/1 -> Terminator/1

== system sim_SS_H2DF_2024a_GRU/dynamics/pre_processing/normalize_last_outputs_MC ==
  data_in : Inport
  Constant : Constant  Value=C2C_NMPC.Normalization.outputs.mean(1)
  Constant1 : Constant  Value=C2C_NMPC.Normalization.outputs.mean(2)
  Constant2 : Constant  Value=C2C_NMPC.Normalization.outputs.mean(3)
  Constant3 : Constant  Value=C2C_NMPC.Normalization.outputs.mean(4)
  Demux : Demux
  Gain : Gain  Gain=1/C2C_NMPC.Normalization.outputs.std(1)
  Gain1 : Gain  Gain=1/C2C_NMPC.Normalization.outputs.std(2)
  Gain2 : Gain  Gain=1/C2C_NMPC.Normalization.outputs.std(3)
  Gain3 : Gain  Gain=1/C2C_NMPC.Normalization.outputs.std(4)
  Mux : Mux
  Selector1 : Selector  IndexOptions=Index vector (dialog)  Indices=[1:4]  OutputSizes=1
  Sum{1..3,5} (4 alike) : Sum  Inputs=|+-
  last_outputs_MC : Outport  VectorParamsAs1DForOutWhenUnconnected=off
  wires:
  Demux/2 -> Sum1/1
  Constant2/1 -> Sum2/2
  Sum2/1 -> Gain2/1
  Sum1/1 -> Gain1/1
  Gain3/1 -> Mux/4
  Gain1/1 -> Mux/2
  Constant1/1 -> Sum1/2
  Demux/3 -> Sum2/1
  Gain2/1 -> Mux/3
  Mux/1 -> last_outputs_MC/1
  Constant3/1 -> Sum3/2
  Sum3/1 -> Gain3/1
  Gain/1 -> Mux/1
  Sum5/1 -> Gain/1
  Constant/1 -> Sum5/2
  Demux/1 -> Sum5/1
  data_in/1 -> Selector1/1
  Demux/4 -> Sum3/1
  Selector1/1 -> Demux/1

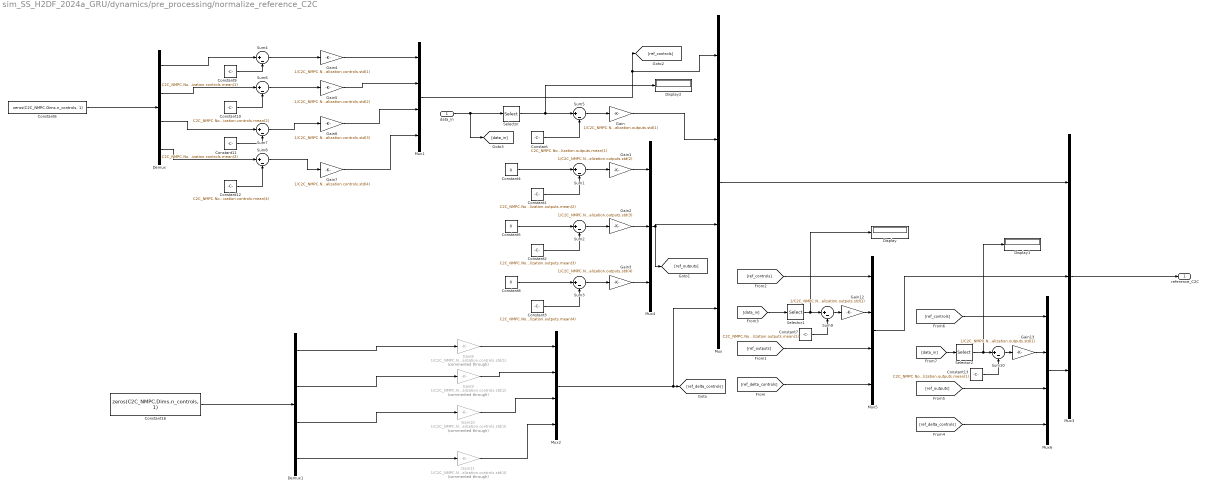
== system sim_SS_H2DF_2024a_GRU/dynamics/pre_processing/normalize_reference_C2C ==
  data_in : Inport
  Constant : Constant  Value=C2C_NMPC.Normalization.outputs.mean(1)
  Constant1 : Constant  Value=C2C_NMPC.Normalization.outputs.mean(2)
  Constant10 : Constant  Value=C2C_NMPC.Normalization.controls.mean(2)
  Constant11 : Constant  Value=C2C_NMPC.Normalization.controls.mean(3)
  Constant12 : Constant  Value=C2C_NMPC.Normalization.controls.mean(4)
  Constant13 : Constant  Value=C2C_NMPC.Normalization.outputs.mean(1)
  Constant16 : Constant  Value=zeros(C2C_NMPC.Dims.n_controls, 1)
  Constant2 : Constant  Value=C2C_NMPC.Normalization.outputs.mean(3)
  Constant3 : Constant  Value=C2C_NMPC.Normalization.outputs.mean(4)
  Constant4 : Constant  Value=0
  Constant5 : Constant  Value=0
  Constant6 : Constant  Value=zeros(C2C_NMPC.Dims.n_controls, 1)
  Constant7 : Constant  Value=C2C_NMPC.Normalization.outputs.mean(1)
  Constant8 : Constant  Value=0
  Constant9 : Constant  Value=C2C_NMPC.Normalization.controls.mean(1)
  Demux : Demux
  Demux1 : Demux
  Display : Display
  Display1 : Display
  Display2 : Display
  Gain : Gain  Gain=1/C2C_NMPC.Normalization.outputs.std(1)
  Gain1 : Gain  Gain=1/C2C_NMPC.Normalization.outputs.std(2)
  Gain10 : Gain  Commented=through  Gain=1/C2C_NMPC.Normalization.controls.std(3)
  Gain11 : Gain  Commented=through  Gain=1/C2C_NMPC.Normalization.controls.std(4)
  Gain12 : Gain  Gain=1/C2C_NMPC.Normalization.outputs.std(1)
  Gain13 : Gain  Gain=1/C2C_NMPC.Normalization.outputs.std(1)
  Gain2 : Gain  Gain=1/C2C_NMPC.Normalization.outputs.std(3)
  Gain3 : Gain  Gain=1/C2C_NMPC.Normalization.outputs.std(4)
  Gain4 : Gain  Gain=1/C2C_NMPC.Normalization.controls.std(1)
  Gain5 : Gain  Gain=1/C2C_NMPC.Normalization.controls.std(2)
  Gain6 : Gain  Gain=1/C2C_NMPC.Normalization.controls.std(3)
  Gain7 : Gain  Gain=1/C2C_NMPC.Normalization.controls.std(4)
  Gain8 : Gain  Commented=through  Gain=1/C2C_NMPC.Normalization.controls.std(1)
  Gain9 : Gain  Commented=through  Gain=1/C2C_NMPC.Normalization.controls.std(2)
  Mux{,1..2,5..6} (5 alike) : Mux
  Mux3 : Mux  Inputs=3
  Mux4 : Mux  Inputs=3
  Selector : Selector  IndexOptions=Index vector (dialog)  Indices=[5]  OutputSizes=1
  Selector1 : Selector  IndexOptions=Index vector (dialog)  Indices=[C2C_NMPC.Dims.n_cost+5]  OutputSizes=1
  Selector2 : Selector  IndexOptions=Index vector (dialog)  Indices=[(C2C_NMPC.Dims.n_cost*2)+5]  OutputSizes=1
  Sum{1..10} (10 alike) : Sum  Inputs=|+-
  reference_C2C : Outport  VectorParamsAs1DForOutWhenUnconnected=off
  wires:
  Constant/1 -> Sum5/2
  data_in/1 -> [data_in], Selector/1
  Sum5/1 -> Gain/1
  Selector/1 -> Display2/1, Sum5/1
  Constant4/1 -> Sum1/1
  Sum1/1 -> Gain1/1
  Constant1/1 -> Sum1/2
  Constant5/1 -> Sum2/1
  Sum2/1 -> Gain2/1
  Constant2/1 -> Sum2/2
  Constant8/1 -> Sum3/1
  Sum3/1 -> Gain3/1
  Constant3/1 -> Sum3/2
  Demux/1 -> Sum4/1
  Sum4/1 -> Gain4/1
  Constant9/1 -> Sum4/2
  Constant6/1 -> Demux/1
  Demux/2 -> Sum6/1
  Constant10/1 -> Sum6/2
  Sum6/1 -> Gain5/1
  Gain5/1 -> Mux1/2
  Gain4/1 -> Mux1/1
  Sum7/1 -> Gain6/1
  Constant11/1 -> Sum7/2
  Demux/3 -> Sum7/1
  Constant12/1 -> Sum8/2
  Sum8/1 -> Gain7/1
  Demux/4 -> Sum8/1
  Gain7/1 -> Mux1/4
  Gain6/1 -> Mux1/3
  Gain9/1 -> Mux2/2
  Gain11/1 -> Mux2/4
  Constant16/1 -> Demux1/1
  Gain8/1 -> Mux2/1
  Gain10/1 -> Mux2/3
  Demux1/4 -> Gain11/1
  Demux1/3 -> Gain10/1
  Demux1/2 -> Gain9/1
  Demux1/1 -> Gain8/1
  Mux2/1 -> [ref_delta_controls], Mux/4
  Mux3/1 -> reference_C2C/1
  Mux/1 -> Mux3/1
  Gain1/1 -> Mux4/1
  Gain2/1 -> Mux4/2
  Gain3/1 -> Mux4/3
  Gain/1 -> Mux/2
  Mux4/1 -> Mux/3, [ref_outputs]
  [ref_delta_controls] -> Mux5/4
  [ref_outputs] -> Mux5/3
  Mux1/1 -> [ref_controls], Mux/1
  [ref_controls] -> Mux5/1
  [data_in] -> Selector1/1
  Mux5/1 -> Mux3/2
  [data_in] -> Selector2/1
  [ref_controls] -> Mux6/1
  [ref_outputs] -> Mux6/3
  [ref_delta_controls] -> Mux6/4
  Mux6/1 -> Mux3/3
  Selector1/1 -> Display/1, Sum9/1
  Sum9/1 -> Gain12/1
  Constant7/1 -> Sum9/2
  Gain12/1 -> Mux5/2
  Constant13/1 -> Sum10/2
  Sum10/1 -> Gain13/1
  Selector2/1 -> Display1/1, Sum10/1
  Gain13/1 -> Mux6/2

== system sim_SS_H2DF_2024a_GRU/reference/reference_dynamic/reference_dynamic ==
  Add1 : Sum
  Clock : Clock
  Constant : Constant
  Constant1 : Constant  Value=[C2C_NMPC.controls_ref;C2C_NMPC.outputs_ref; zeros(C2C_NMPC.Dims.n_controls, length(C2C_NMPC.controls_ref(1, :)))]
  ref_func : MATLAB Function  InitFcn=|  TreatAsAtomicUnit=on
      | cost_length = C2C_NMPC.Dims.n_cost ;
      | horizon_length = 3;
      | %C2C_NMPC.Opts.N; 
      | y_ref_buf = zeros(cost_length, horizon_length);
  reference : Outport  VectorParamsAs1DForOutWhenUnconnected=off
  wires:
  Clock/1 -> Add1/1
  Add1/1 -> ref_func/2(init_index)
  Constant/1 -> Add1/2
  Constant1/1 -> ref_func/1(ref_norm)
  ref_func/1(y_ref) -> reference/1
